simulink model "Advanced_PID_with_OPC"  (R2023a)
settings: Solver=VariableStepAuto  StartTime=0.0  StopTime=inf  RelTol=1e-3
model workspace (MAT data in the model file):
  A = [400000 0]
  Ti = 0
libraries: opclib x4, slpidlib x1
settings Model: PacingRate=5  Creator=munam  LastModifiedBy=Yuganshu Wadhwa

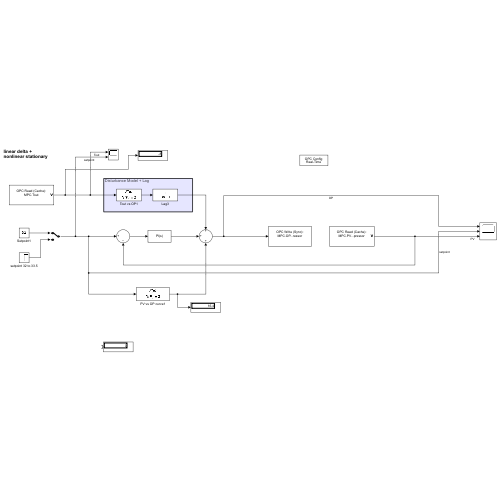
[thumbnail: Simulink's stored preview of the top-level diagram]
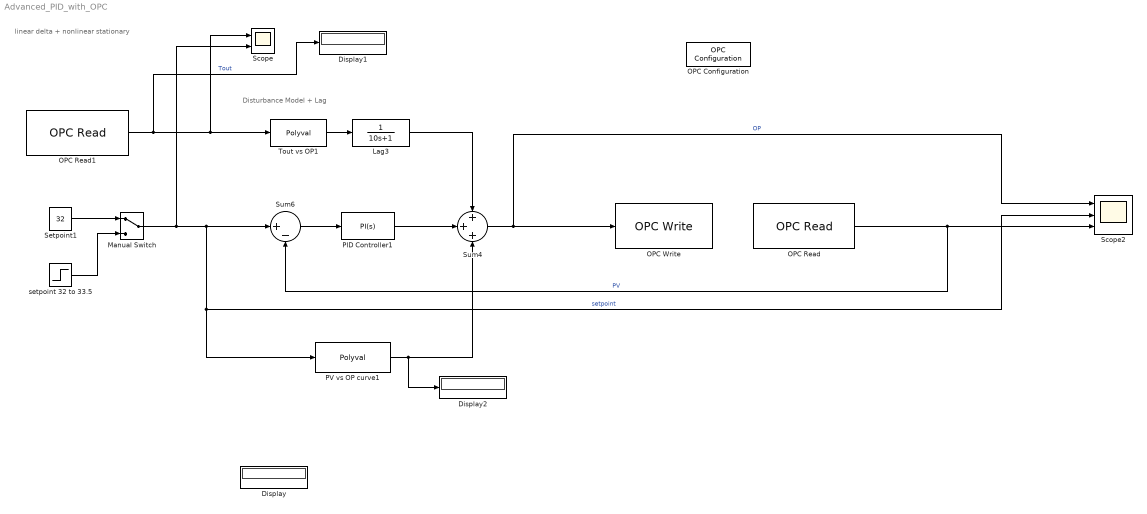
== system Advanced_PID_with_OPC ==
  note: Disturbance Model + Lag
  note: linear delta + nonlinear stationary
  Display : Display
  Display1 : Display
  Display2 : Display
  Lag3 : TransferFcn  Denominator=[10 1]
  Manual Switch : ManualSwitch
  OPC Configuration : opclib/OPC Configuration  opcServers=localhost/Matrikon.OPC.Simulation.1/10  errMissingItems=Error  errReadWrite=Warn  errShutdown=Error  errRTViolation=Warn  rtEnable=on  speedup=1  showLatency=off  beingUsed=on
  OPC Read : opclib/OPC Read  serverHost=localhost  serverID=Matrikon.OPC.Simulation.1  itemIDs=MPC.PV_Compressor  readMode=Synchronous (cache)  dataType=double  updateRate=0.5  showQual=off  showTS=off  tsMode=Seconds since start
  OPC Read1 : opclib/OPC Read  serverHost=localhost  serverID=Matrikon.OPC.Simulation.1  itemIDs=MPC.Tout  readMode=Synchronous (cache)  dataType=double  updateRate=0.5  showQual=off  showTS=off  tsMode=Seconds since start
  OPC Write : opclib/OPC Write  serverHost=localhost  serverID=Matrikon.OPC.Simulation.1  itemIDs=MPC.OP_Compressor  writeMode=Synchronous  updateRate=0
  PID Controller1 : slpidlib/PID Controller  Controller=PI  Form=Parallel  TimeDomain=Continuous-time  UseExternalTs=off  SampleTime=-1  IntegratorMethod=Forward Euler  FilterMethod=Forward Euler  ControllerParametersSource=internal  P=3  I=1  UseKiTs=off  D=0  N=1  UseFilter=on  TunerSelectOption=Transfer Function Based (PID Tuner App)  InitialConditionSource=internal  InitialConditionForIntegrator=0  InitialConditionForFilter=0  DifferentiatorICPrevScaledInput=0  ExternalReset=none  TrackingMode=off  Kt=1  LimitOutput=off  SatLimitsSource=internal  UpperSaturationLimit=100  LowerSaturationLimit=0  LinearizeAsGain=off  AntiWindupMode=back-calculation  Kb=1  LimitIntegrator=off  UpperIntegratorSaturationLimit=inf  LowerIntegratorSaturationLimit=-inf  POutMin=[]  POutMax=[]  IOutMin=[]  IOutMax=[]  DOutMin=[]  DOutMax=[]  NOutMin=[]  NOutMax=[]  SumOutMin=[]  SumOutMax=[]  SaturationOutMin=[]  SaturationOutMax=[]  PParamMin=[]  PParamMax=[]  IParamMin=[]  IParamMax=[]  DParamMin=[]  DParamMax=[]  NParamMin=[]  NParamMax=[]  KbParamMin=[]  KbParamMax=[]  KtParamMin=[]  KtParamMax=[]  KbOutMin=[]  KbOutMax=[]  KtOutMin=[]  KtOutMax=[]  IntegratorOutMin=[]  IntegratorOutMax=[]  FilterOutMin=[]  FilterOutMax=[]  SumI1OutMin=[]  SumI1OutMax=[]  SumI2OutMin=[]  SumI2OutMax=[]  SumI3OutMin=[]  SumI3OutMax=[]  SumI4OutMin=[]  SumI4OutMax=[]  SumDOutMin=[]  SumDOutMax=[]  DifferentiatorOutMin=[]  DifferentiatorOutMax=[]  FilterDiffOutCoefMin=[]  FilterDiffOutCoefMax=[]  ReciprocalOutMin=[]  ReciprocalOutMax=[]  SumDenOutMin=[]  SumDenOutMax=[]  SumNumOutMin=[]  SumNumOutMax=[]  DivideOutMin=[]  DivideOutMax=[]  UdiffTsProdOutMin=[]  UdiffTsProdOutMax=[]  NTsProdOutMin=[]  NTsProdOutMax=[]  UintegralTsProdOutMin=[]  UintegralTsProdOutMax=[]  UngainTsProdOutMin=[]  UngainTsProdOutMax=[]  ClampingZeroOutDataTypeStr=Inherit: Inherit via back propagation  ClampingZeroOutMin=[]  ClampingZeroOutMax=[]  FilterDenConstantOutDataTypeStr=Inherit: Inherit via back propagation  FilterDenConstantOutMin=[]  FilterDenConstantOutMax=[]  PCopyOutDataTypeStr=Inherit: Inherit via back propagation  PCopyOutMin=[]  PCopyOutMax=[]  NCopyOutDataTypeStr=Inherit: Inherit via back propagation  NCopyOutMin=[]  NCopyOutMax=[]  IntegratorContinuousStateAttributes=''  IntegratorStateMustResolveToSignalObject=off  IntegratorRTWStateStorageClass=Auto  FilterContinuousStateAttributes=''  FilterStateMustResolveToSignalObject=off  FilterRTWStateStorageClass=Auto  ParallelPVariant=InternalParameters  IdealPVariant=Disabled  IVariant=InternalParameters  DVariant=Disabled  IntegratorVariant=Continuous  SatVariant=Disabled  AWVariant=Passthrough  PCopyVariant=Disabled  TRVariant=Disabled  FdbkBlocksVariant=Forward  IdealPFdbkVariant=Disabled  SatFdbkVariant=Disabled  DerivativeFilterVariant=Disabled  NVariant=Disabled  NCopyVariant=Disabled_SignalSpec  FilterICVariant=Disabled  IntegratorICVariant=InternalICs  ExternalResetVariant=Disabled  TRSumVariant=Passthrough  SumFdbkVariant=Disabled  SumVariant=Sum_PI  TsampFilterVariant=InternalTs  TsampNgainVariant=Passthrough  TsampIntegralVariant=Disabled_SignalSpec  ExternalSaturationOutDataTypeStr=Inherit: Same as second input
  PV vs OP curve1 : Polyval  Coefs=[ +20.075, -1284.7, 20570]
  Scope : Scope  NumInputPorts=2
  Scope2 : Scope  NumInputPorts=3
  Setpoint1 : Constant  Value=32
  Sum4 : Sum  Inputs=+++
  Sum6 : Sum  Inputs=|+-
  Tout vs OP1 : Polyval  Coefs=[ +0.5285, +0.2364, +16.302 ]
  setpoint 32 to 33.5 : Step  Time=100  Before=32  After=33.5  SampleTime=0
  wires:
  PV vs OP curve1/1 -> Display2/1, Sum4/3
  Manual Switch/1 -> Scope/2, PV vs OP curve1/1, Scope2/2, Sum6/1  "setpoint"
  OPC Read/1 -> Scope2/3, Sum6/2  "PV"
  PID Controller1/1 -> Sum4/2
  OPC Read1/1 -> Display1/1, Scope/1, Tout vs OP1/1  "Tout"
  Sum6/1 -> PID Controller1/1
  Tout vs OP1/1 -> Lag3/1
  Sum4/1 -> OPC Write/1, Scope2/1  "OP"
  Lag3/1 -> Sum4/1
  Setpoint1/1 -> Manual Switch/1
  setpoint 32 to 33.5/1 -> Manual Switch/2
